simulink model "a1"  (R2022b)
settings: Solver=VariableStepAuto  StartTime=0.0  StopTime=20  FixedStep=0.001  MaxStep=Auto  MinStep=Auto  RelTol=1e-3
values from neighbouring files (symbols this model uses):
  Astate = [A1; A2; A3; A4; A5; A6]    [AME556_HW4_Cornwell.m]    (also in AME_556_Final_Project.m)
  calfd = -1.6    [AME556_HW3_Cornwell.m]    (also in AME_556_Final_Project.m)
  dt = params.dt    [AME556_HW4_Cornwell.m]    (also in AME_556_Final_Project.m = 0.03)
  gait_type = 1    [AME_556_Final_Project.m]
  H = H3    [AME556_HW1_Cornwell.m]    (also in AME556_HW4_Cornwell.m = blkdiag(H,Rmpc); AME_556_Final_Project.m = blkdiag(H,Rmpc))
  hipd = 0    [AME556_HW3_Cornwell.m]    (also in AME_556_Final_Project.m)
  kd = params.kd    [AME556_HW3_Cornwell.m]    (also in AME_556_Final_Project.m = 4)
  kp = params.kp    [AME556_HW3_Cornwell.m]    (also in AME_556_Final_Project.m = 25)
  m = params.m    [AME556_HW3_Cornwell.m]    (also in AME556_HW4_Cornwell.m = params.mass)
  N = size(x, 2)    [AME556_HW3_Cornwell.m]    (also in AME556_HW4_Cornwell.m; AME_556_Final_Project.m = 10)
  PD = 0    [AME_556_Final_Project.m]
  Q = diag([40 50 60 10 10 10 4 4 4 1 1 1 0])    [AME556_HW4_Cornwell.m]    (also in AME_556_Final_Project.m = diag([0 800 15000 49500 14000 5000 1900 700 700 900 700 200 )
  speed = 0.37    [AME_556_Final_Project.m]
  thighd = 0.95    [AME556_HW3_Cornwell.m]    (also in AME_556_Final_Project.m)
  Tstance = 0.15    [AME_556_Final_Project.m]
  X = quadprog(H,f,Astate,bstate,Aeq,beq)    [AME556_HW4_Cornwell.m]
  z0 = [x0(1)-1; x0(2)]    [AME556_HW5_Cornwell.m]    (also in AME_556_Final_Project.m = 0.2855)
  zd = 0.31    [AME_556_Final_Project.m]
undefined symbols (not defined in the file or in its folder): Y, Z
libraries: sm_lib x181, nesl_utility x96
(part 6 of 6)

== matlab function a1/Convert to torque ==
  settings: sampleTime=0.001
  data: J_FL input; J_FR input; J_RL input; J_RR input; gait_type input; tau input; PD input; x input; u_MPC input; u_FP input; u_QP input; t_FL output; t_FR output; t_RL output; t_RR output; gait_table input
function [t_FL, t_FR, t_RL, t_RR] = fcn(J_FL, J_FR, J_RL, J_RR, gait_type,...
    tau, PD, x, u_MPC, u_FP, u_QP, gait_table)

    % Rotation matrix from x
    R = eul2rotm([x(6),x(5),x(4)]);

    % Tau from PD controller


    % Initialize
    F1 = zeros(3,1);
    F2 = zeros(3,1);
    F3 = zeros(3,1);
    F4 = zeros(3,1);
    
    % Check if each foot is in stance (MPC) or swing (FP)
    if gait_type == 0
        if PD == 0
            F1(1:3,1) = u_QP(1:3);
            t_FL = -transpose(J_FL)*transpose(R)*F1;    % 1
        else
            t_FL = [tau(1);tau(2);tau(3)];
        end
    elseif gait_table(1,1) == 1 
        F1(1:3,1) = u_MPC(1:3);
        t_FL = -transpose(J_FL)*transpose(R)*F1;    % 1
    else
        F1(1:3,1) = u_FP(1:3);
        t_FL = transpose(J_FL)*transpose(R)*F1;    % 1
    end

    if gait_type == 0
        if PD == 0
            F2(1:3,1) = u_QP(4:6);
            t_FR = -transpose(J_FR)*transpose(R)*F2;    % 2
        else
            t_FR = [tau(4);tau(5);tau(6)];
        end
    elseif gait_table(2,1) == 1
        F2(1:3,1) = u_MPC(4:6);
        t_FR = -transpose(J_FR)*transpose(R)*F2;    % 2
    else
        F2(1:3,1) = u_FP(4:6);
        t_FR = transpose(J_FR)*transpose(R)*F2;    % 2
    end
    
    if gait_type == 0
        if PD == 0
            F3(1:3,1) = u_QP(7:9);
            t_RL = -transpose(J_RL)*transpose(R)*F3;    % 3
        else
            t_RL = [tau(7);tau(8);tau(9)];
        end
    elseif gait_table(3,1) == 1
        F3(1:3,1) = u_MPC(7:9);
        t_RL = -transpose(J_RL)*transpose(R)*F3;    % 3
    else
        F3(1:3,1) = u_FP(7:9);
        t_RL = transpose(J_RL)*transpose(R)*F3;    % 3
    end

    if gait_type == 0
        if PD == 0
            F4(1:3,1) = u_QP(10:12);
            t_RR = -transpose(J_RR)*transpose(R)*F4;    % 4
        else
            t_RR = [tau(10);tau(11);tau(12)];
        end
    elseif gait_table(4,1) == 1
        F4(1:3,1) = u_MPC(10:12);
        t_RR = -transpose(J_RR)*transpose(R)*F4;    % 4
    else
        F4(1:3,1) = u_FP(10:12);
        t_RR = transpose(J_RR)*transpose(R)*F4;    % 4
    end

end

== matlab function a1/MPC and QP/MPC controller ==
  settings: updateMethod=DISCRETE  sampleTime=dt
  data: x input; pf input; N input; dt input; H input; Q input; Astate input; Xd input; gait_table input; gait_type input; u output
% MPC gait controller
function u = MPC_gait(x,pf,N,dt,H,Q,Astate,Xd,gait_table,gait_type)
    if gait_type == 0 % standing w/ QP
        u = zeros(12,1); % do not use MPC
    else
        % N = number of horizons
        % dt = sampling times in s
        % gait_table = matrix with stance/swing values for each iteration
    
        % Robot parameters
        mass = 12;
        I = diag([0.0168, 0.0565, 0.064]);

        % Foot positions
        pf_FL = [pf(1);pf(2);pf(3)];
        pf_FR = [pf(4);pf(5);pf(6)];
        pf_RL = [pf(7);pf(8);pf(9)];
        pf_RR = [pf(10);pf(11);pf(12)];

        % Rearrange to get x_bar
        px = x(1); py = x(2); pz = x(3);
        p = [px;py;pz];

        roll = x(4); pitch = x(5); yaw = x(6);
        theta = [roll; pitch; yaw];

        dx = x(7); dy = x(8); dz = x(9);
        dp = [dx;dy;dz];
        
        wx = x(10); wy = x(11); wz = x(12);
        w = [wx;wy;wz];
    
        % Control input
        x_bar = [p; theta; dp; w; -9.81];
    
        % Controller settings
        f = -transpose([repmat(transpose(Xd)*Q,1,N) zeros(1,12*N)]);
    
        % dtheta
        T = [cos(yaw)*cos(0), -sin(yaw), 0;
             sin(yaw)*cos(0), cos(yaw), 0;
             -sin(0), 0, 1];
    
        % Make continuous --> discrete dynamics: dX = AX + Bu
        Acont = [zeros(3,6) eye(3) zeros(3,4);
                 zeros(3,9) inv(T) zeros(3,1);
                 zeros(2,13);
                 zeros(1,12) 1;
                 zeros(4,13)]; % (13x13)
    
        % r vectors in world frame
        r1 = pf_FL - p; % ri = pf-p
        r2 = pf_FR - p;
        r3 = pf_RL - p;
        r4 = pf_RR - p;
    
        r1x = [0, -r1(3), r1(2);
               r1(3), 0, -r1(1);
               -r1(2), r1(1), 0];
        r2x = [0, -r2(3), r2(2);
               r2(3), 0, -r2(1);
               -r2(2), r2(1), 0];
        r3x = [0, -r3(3), r3(2);
               r3(3), 0, -r3(1);
               -r3(2), r3(1), 0];
        r4x = [0, -r4(3), r4(2);
               r4(3), 0, -r4(1);
               -r4(2), r4(1), 0];
    
        Bcont = [zeros(6,12);
                 eye(3)./mass eye(3)./mass eye(3)./mass eye(3)./mass;
                 I\r1x, I\r2x, I\r3x, I\r4x;
                 zeros(1,12)]; % (13x12)
    
        A = Acont.*dt+eye(13);
        B = Bcont.*dt;
    
        % State-dependent constraints: AX <= b
        % Fz constraints
%         b = [500; 500; 500; 500];
%         b1 = repmat(b,N,1);
        b1 = zeros(4*N,1);
        for i = 0:N-1
            for j = 1:4
                b1(4*i + j,1) = 500*gait_table(4*i + j);
            end
        end
        b2 = b1./(-50);
    
        % Fx/Fz constraints
        b = [0; 0; 0; 0];
        b3 = repmat(b,N,1);
        b4 = b3;
    
        % Fy/Fz constraints
        b5 = b3;
        b6 = b3;
    
        bstate = [b1; b2; b3; b4; b5; b6];
    
        % Equality constraints
        Aeq = zeros(13*N,25*N);               % (13N,25N)
        for ii = 1:N
            Aeq(13*(ii-1)+1:13*ii,13*(ii-1)+1:13*ii) = eye(13,13);
            if ii > 1
                Aeq(13*(ii-1)+1:13*ii,13*(ii-2)+1:13*(ii-1)) = -A;
            end
            Aeq(13*(ii-1)+1:13*ii,13*N+12*(ii-1)+1:13*N+12*ii) = -B;
        end
    
        beq = [A*x_bar; zeros(13*(N-1),1)]; % (13N,1)
        
        % Solve
        options = optimoptions('quadprog','Display','off','Algorithm','active-set'); 
        x0 = zeros(length(H),1);
        X = quadprog(H,f,Astate,bstate,Aeq,beq,[],[],x0,options);
    
        u = zeros(12,1);
        u = X(13*N+1:13*N+12);
    end

end

== matlab function a1/MATLAB Function ==
  data: q input; J output; leg input
function J = computeLegJacobian(q,leg)
     
    l1=0.045; % hip length
%     l1 = 0.0838;
    l2=0.2; % thigh length
    l3=0.2; % calf length
    
    if leg==1 || leg==3 % left leg (FL and RL) has sideSign 1
        sideSign=1;
    else
        sideSign=-1; % right leg (FR and RR) has sideSign -1
    end
    s1=sin(q(1)); % for hip joint
    s2=sin(q(2)); % for thigh joint
    s3=sin(q(3)); % for calf joint
    
    c1=cos(q(1)); % for hip joint
    c2=cos(q(2)); % for thigh joint
    c3=cos(q(3)); % for calf joint
    
    c23=c2*c3-s2*s3;
    s23=s2*c3+c2*s3;
    
    J = zeros(3,3);
    J(1,1)=0;
    J(2,1)=-sideSign*l1*s1+l2*c2*c1+l3*c23*c1;
    J(3,1)=sideSign*l1*c1+l2*c2*s1+l3*c23*s1;
    
    J(1,2)=-l3*c23-l2*c2;
    J(2,2)=-l2*s2*s1-l3*s23*s1;
    J(3,2)=l2*s2*c1+l3*s23*c1;
    
    J(1,3)=-l3*c23;
    J(2,3)=-l3*s23*s1;
    J(3,3)=l3*s23*c1;

end

== matlab function a1/MATLAB Function1 ==
  data: q input; J output; leg input
function J = computeLegJacobian(q,leg)
     
    l1=0.045; % hip length
%     l1 = 0.0838;
    l2=0.2; % thigh length
    l3=0.2; % calf length
    
    if leg==1 || leg==3 % left leg (FL and RL) has sideSign 1
        sideSign=1;
    else
        sideSign=-1; % right leg (FR and RR) has sideSign -1
    end
    s1=sin(q(1)); % for hip joint
    s2=sin(q(2)); % for thigh joint
    s3=sin(q(3)); % for calf joint
    
    c1=cos(q(1)); % for hip joint
    c2=cos(q(2)); % for thigh joint
    c3=cos(q(3)); % for calf joint

    c23=c2*c3-s2*s3;
    s23=s2*c3+c2*s3;
    
    J = zeros(3,3);
    J(1,1)=0;
    J(2,1)=-sideSign*l1*s1+l2*c2*c1+l3*c23*c1;
    J(3,1)=sideSign*l1*c1+l2*c2*s1+l3*c23*s1;
    
    J(1,2)=-l3*c23-l2*c2;
    J(2,2)=-l2*s2*s1-l3*s23*s1;
    J(3,2)=l2*s2*c1+l3*s23*c1;
    
    J(1,3)=-l3*c23;
    J(2,3)=-l3*s23*s1;
    J(3,3)=l3*s23*c1;

end

== matlab function a1/MATLAB Function2 ==
  data: q input; J output; leg input
function J = computeLegJacobian(q,leg)
     
    l1=0.045; % hip length
%     l1 = 0.0838;
    l2=0.2; % thigh length
    l3=0.2; % calf length
    
    if leg==1 || leg==3 % left leg (FL and RL) has sideSign 1
        sideSign=1;
    else
        sideSign=-1; % right leg (FR and RR) has sideSign -1
    end
    s1=sin(q(1)); % for hip joint
    s2=sin(q(2)); % for thigh joint
    s3=sin(q(3)); % for calf joint
    
    c1=cos(q(1)); % for hip joint
    c2=cos(q(2)); % for thigh joint
    c3=cos(q(3)); % for calf joint

    c23=c2*c3-s2*s3;
    s23=s2*c3+c2*s3;
    
    J = zeros(3,3);
    J(1,1)=0;
    J(2,1)=-sideSign*l1*s1+l2*c2*c1+l3*c23*c1;
    J(3,1)=sideSign*l1*c1+l2*c2*s1+l3*c23*s1;
    
    J(1,2)=-l3*c23-l2*c2;
    J(2,2)=-l2*s2*s1-l3*s23*s1;
    J(3,2)=l2*s2*c1+l3*s23*c1;
    
    J(1,3)=-l3*c23;
    J(2,3)=-l3*s23*s1;
    J(3,3)=l3*s23*c1;
end

== matlab function a1/MATLAB Function4 ==
  data: q input; J output; leg input
function J = computeLegJacobian(q,leg)
     
    l1=0.045; % hip length
%     l1 = 0.0838;
    l2=0.2; % thigh length
    l3=0.2; % calf length
    
    if leg==1 || leg==3 % left leg (FL and RL) has sideSign 1
        sideSign=1;
    else
        sideSign=-1; % right leg (FR and RR) has sideSign -1
    end
    s1=sin(q(1)); % for hip joint
    s2=sin(q(2)); % for thigh joint
    s3=sin(q(3)); % for calf joint
    
    c1=cos(q(1)); % for hip joint
    c2=cos(q(2)); % for thigh joint
    c3=cos(q(3)); % for calf joint

    c23=c2*c3-s2*s3;
    s23=s2*c3+c2*s3;
    
    J = zeros(3,3);
    J(1,1)=0;
    J(2,1)=-sideSign*l1*s1+l2*c2*c1+l3*c23*c1;
    J(3,1)=sideSign*l1*c1+l2*c2*s1+l3*c23*s1;
    
    J(1,2)=-l3*c23-l2*c2;
    J(2,2)=-l2*s2*s1-l3*s23*s1;
    J(3,2)=l2*s2*c1+l3*s23*c1;
    
    J(1,3)=-l3*c23;
    J(2,3)=-l3*s23*s1;
    J(3,3)=l3*s23*c1;

end
